simulink model "hw_lab4_1sim"  (R2021b)
settings: Solver=VariableStepAuto  StartTime=0.0  StopTime=10.0  RelTol=1e-3
settings Model: Creator=1412  LastModifiedBy=1412

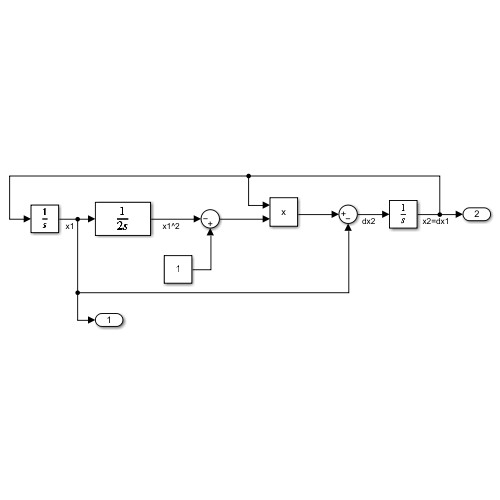
[thumbnail: Simulink's stored preview of the top-level diagram]
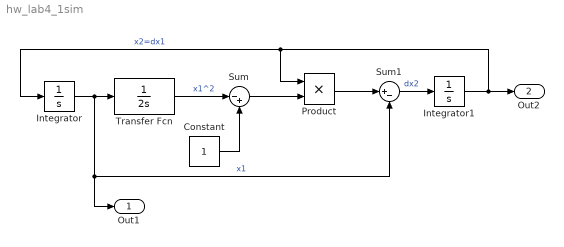
== system hw_lab4_1sim ==
  Constant : Constant
  Integrator : Integrator
  Integrator1 : Integrator
  Product : Product
  Sum : Sum  Inputs=|-+
  Sum1 : Sum  Inputs=|+-
  Transfer Fcn : TransferFcn  Denominator=[2 0]
  Out1 : Outport
  Out2 : Outport  Port=2
  wires:
  Integrator/1 -> Out1/1, Sum1/2, Transfer Fcn/1  "x1"
  Transfer Fcn/1 -> Sum/1  "x1^2"
  Constant/1 -> Sum/2
  Sum/1 -> Product/2
  Product/1 -> Sum1/1
  Sum1/1 -> Integrator1/1  "dx2"
  Integrator1/1 -> Product/1, Integrator/1, Out2/1  "x2=dx1"
